simulink model "systemSimulink"  (R2021a)
settings: Solver=ode45  StartTime=0.0  StopTime=100  RelTol=1e-5
InitFcn:
  | setupSimulink
StopFcn:
  | resultPlot
values from neighbouring files (symbols this model uses):
  K1 = 100    [setupSimulink.m]
  K2 = 500    [setupSimulink.m]
  Kp = 0.8    [setupSimulink.m]
undefined symbols (not defined in the file or in its folder): fPWM_I1, fPWM_V2
settings Model: Creator=alfy  LastModifiedBy=alfy

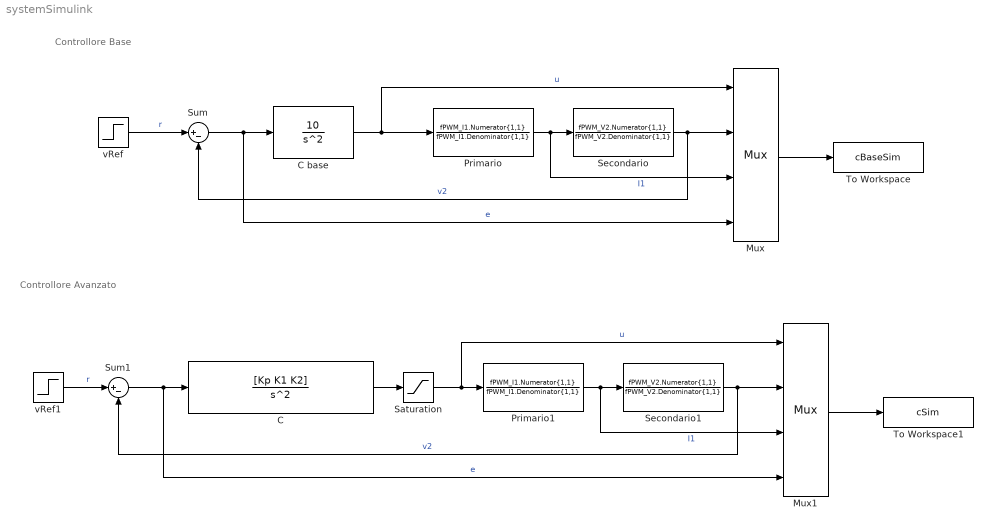
== system systemSimulink ==
  note: Controllore Avanzato
  note: Controllore Base
  C : TransferFcn  Numerator=[Kp K1 K2]  Denominator=[ 1 0 0]
  C base : TransferFcn  Numerator=[10]  Denominator=[1 0 0]
  Mux : Mux
      settings: DisplayOption=signals
  Mux1 : Mux
      settings: DisplayOption=signals
  Primario : TransferFcn  Numerator=fPWM_I1.Numerator{1,1}  Denominator=fPWM_I1.Denominator{1,1}
  Primario1 : TransferFcn  Numerator=fPWM_I1.Numerator{1,1}  Denominator=fPWM_I1.Denominator{1,1}
  Saturation : Saturate  UpperLimit=1  LowerLimit=-1
  Secondario : TransferFcn  Numerator=fPWM_V2.Numerator{1,1}  Denominator=fPWM_V2.Denominator{1,1}
  Secondario1 : TransferFcn  Numerator=fPWM_V2.Numerator{1,1}  Denominator=fPWM_V2.Denominator{1,1}
  Sum : Sum  Inputs=|+-
  Sum1 : Sum  Inputs=|+-
  To Workspace : ToWorkspace  VariableName=cBaseSim  SaveFormat=Structure With Time  SampleTime=-1
  To Workspace1 : ToWorkspace  VariableName=cSim  SaveFormat=Structure With Time  SampleTime=-1
  vRef : Step  Time=0.3  After=0.5  SampleTime=0
  vRef1 : Step  Time=0.3  After=0.5  SampleTime=0
  wires:
  Sum/1 -> Mux/4, C base/1  "e"
  vRef/1 -> Sum/1  "r"
  Secondario/1 -> Sum/2, Mux/2  "v2"
  Mux/1 -> To Workspace/1
  Primario/1 -> Mux/3, Secondario/1  "I1"
  C base/1 -> Primario/1, Mux/1  "u"
  vRef1/1 -> Sum1/1  "r"
  Mux1/1 -> To Workspace1/1
  Primario1/1 -> Mux1/3, Secondario1/1  "I1"
  Sum1/1 -> C/1, Mux1/4  "e"
  C/1 -> Saturation/1
  Secondario1/1 -> Sum1/2, Mux1/2  "v2"
  Saturation/1 -> Mux1/1, Primario1/1  "u"
